simulink model "dc_motor"  (R2024b)
settings: Solver=VariableStepAuto  StartTime=0.0  StopTime=10.0  RelTol=1e-3
settings Model: Creator=Admin  LastModifiedBy=pragy

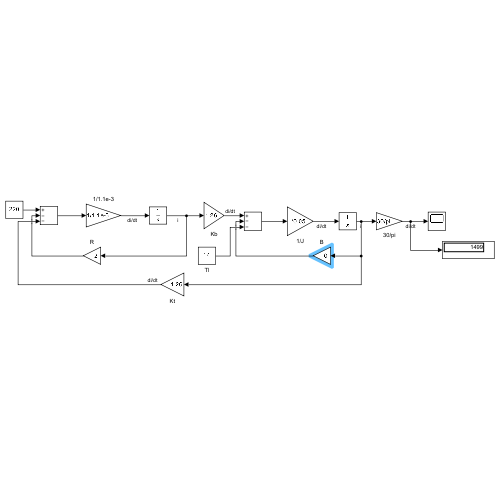
[thumbnail: Simulink's stored preview of the top-level diagram]
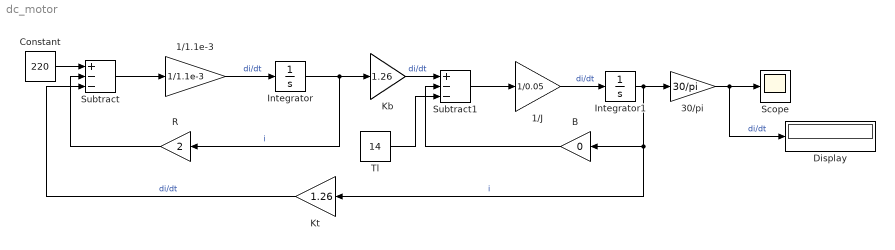
== system dc_motor ==
  1/1.1e-3 : Gain  Gain=1/1.1e-3
  1/J : Gain  Gain=1/0.05
  30/pi : Gain  Gain=30/pi
  B : Gain  Gain=0
  Constant : Constant  Value=220
  Display : Display
  Integrator : Integrator
  Integrator1 : Integrator
  Kb : Gain  Gain=1.26
  Kt : Gain  Gain=1.26
  R : Gain  Gain=2
  Scope : Scope
  Subtract : Sum  Inputs=+--
  Subtract1 : Sum  Inputs=+--
  Tl : Constant  Value=14
  wires:
  Integrator/1 -> Kb/1, R/1  "i"
  Subtract/1 -> 1/1.1e-3/1
  R/1 -> Subtract/2
  Constant/1 -> Subtract/1
  1/1.1e-3/1 -> Integrator/1  "di/dt"
  Kb/1 -> Subtract1/1  "di/dt"
  Tl/1 -> Subtract1/3
  B/1 -> Subtract1/2
  Subtract1/1 -> 1/J/1
  1/J/1 -> Integrator1/1  "di/dt"
  Integrator1/1 -> 30/pi/1, B/1, Kt/1  "i"
  30/pi/1 -> Display/1, Scope/1  "di/dt"
  Kt/1 -> Subtract/3  "di/dt"
